simulink model "simu"  (R2023b)
settings: Solver=VariableStepAuto  StartTime=0.0  StopTime=1  RelTol=1e-3
values from neighbouring files (symbols this model uses):
  J = J_r+J_m+J_d    (= 2.15e-05)    [K_calculator.m]    (also in Velocity.m; mappe2.m)
  K_b = 0.042    [K_calculator.m]    (also in Velocity.m; mappe2.m)
  K_t = 0.042    [K_calculator.m]    (also in Velocity.m; mappe2.m)
  R_a = 8.4    [K_calculator.m]    (also in Velocity.m; mappe2.m)
settings Model: Creator=vegar  LastModifiedBy=vegar

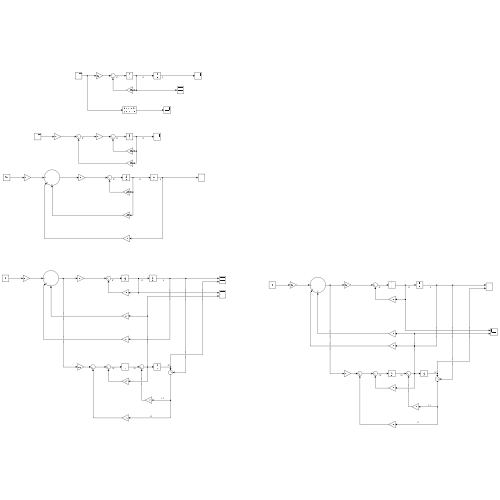
[thumbnail: Simulink's stored preview of the top-level diagram]
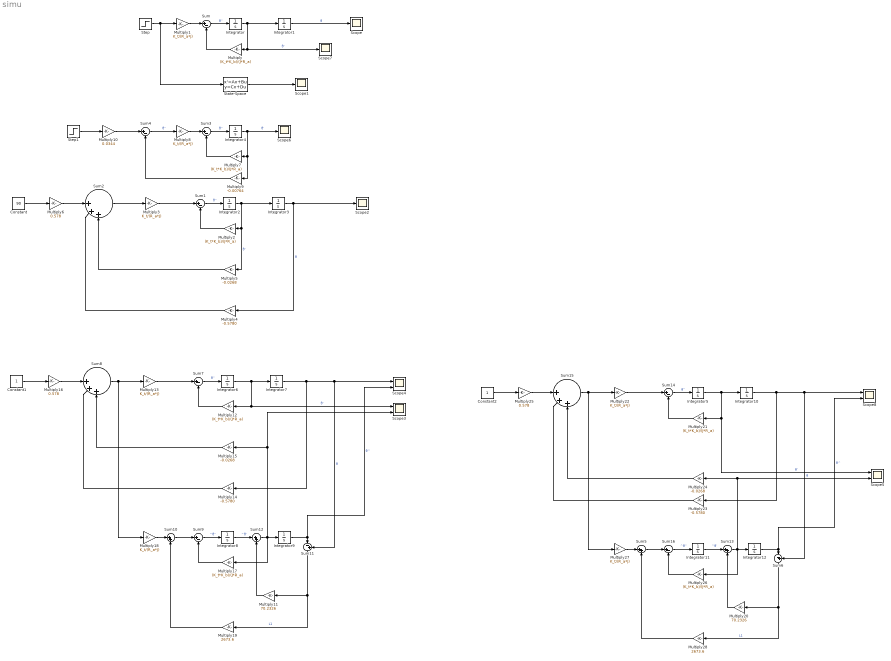
== system simu ==
  Constant : Constant  Value=90
  Constant1 : Constant
  Constant2 : Constant
  Integrator{,1..2,4..6,8..9,11..12} (10 alike) : Integrator
  Integrator10 : Integrator  InitialCondition=30
  Integrator3 : Integrator  InitialCondition=0.1
  Integrator7 : Integrator  InitialCondition=30
  Multiply{,2,7,12,17,21,26} (7 alike) : Gain  Gain=(K_t*K_b)/(J*R_a)
  Multiply{1,3,8,13,18,22,27} (7 alike) : Gain  Gain=K_t/(R_a*J)
  Multiply10 : Gain  Gain=0.0344
  Multiply11 : Gain  Gain=70.2326
  Multiply14 : Gain  Gain=-0.5780
  Multiply15 : Gain  Gain=-0.0268
  Multiply16 : Gain  Gain=0.578
  Multiply19 : Gain  Gain=2673.6
  Multiply20 : Gain  Gain=70.2326
  Multiply23 : Gain  Gain=-0.5780
  Multiply24 : Gain  Gain=-0.0268
  Multiply25 : Gain  Gain=0.578
  Multiply28 : Gain  Gain=2673.6
  Multiply4 : Gain  Gain=-0.5780
  Multiply5 : Gain  Gain=-0.0268
  Multiply6 : Gain  Gain=0.578
  Multiply9 : Gain  Gain=-0.00764
  Scope{,1..2,6..7} (5 alike) : Scope
  Scope{3..5,8} (4 alike) : Scope  NumInputPorts=2
  State-Space : StateSpace  A=[0 1; 0 -(K_t*K_b)/(J*R_a)]  B=[0;K_t/(R_a*J)]  C=[1 0]  D=0  InitialCondition=0
  Step : Step  SampleTime=0
  Step1 : Step  After=203  SampleTime=0
  Sum{,1,3..4,7,9,14,16} (8 alike) : Sum  Inputs=|+-
  Sum{5,10,12..13} (4 alike) : Sum  Inputs=|++
  Sum11 : Sum  Inputs=|-+
  Sum15 : Sum  Inputs=||+++
  Sum2 : Sum  Inputs=||+++
  Sum6 : Sum  Inputs=|-+
  Sum8 : Sum  Inputs=||+++
  wires:
  Integrator1/1 -> Scope/1  "θ"
  Integrator/1 -> Integrator1/1, Scope7/1, Multiply/1  "θ'"
  Sum/1 -> Integrator/1  "θ''"
  Step/1 -> Multiply1/1, State-Space/1
  Multiply/1 -> Sum/2
  State-Space/1 -> Scope1/1
  Sum1/1 -> Integrator2/1  "θ''"
  Multiply2/1 -> Sum1/2
  Integrator2/1 -> Multiply2/1, Multiply5/1, Integrator3/1  "θ'"
  Integrator3/1 -> Scope2/1, Multiply4/1  "θ"
  Multiply4/1 -> Sum2/2
  Multiply5/1 -> Sum2/3
  Constant/1 -> Multiply6/1
  Sum2/1 -> Multiply3/1
  Multiply6/1 -> Sum2/1
  Multiply3/1 -> Sum1/1
  Multiply19/1 -> Sum10/2
  Sum10/1 -> Sum9/1
  Multiply18/1 -> Sum10/1
  Multiply11/1 -> Sum12/2
  Sum11/1 -> Multiply11/1, Multiply19/1  "L1"
  Multiply13/1 -> Sum7/1
  Sum12/1 -> Multiply15/1, Scope3/2, Multiply17/1, Integrator9/1
  Multiply16/1 -> Sum8/1
  Integrator9/1 -> Scope4/2, Sum11/1  "θ^"
  Sum9/1 -> Integrator8/1  "^θ''"
  Integrator7/1 -> Scope4/1, Sum11/2, Multiply14/1  "θ"
  Integrator8/1 -> Sum12/1  "^θ'"
  Multiply12/1 -> Sum7/2
  Constant1/1 -> Multiply16/1
  Integrator6/1 -> Integrator7/1, Scope3/1, Multiply12/1  "θ'"
  Multiply14/1 -> Sum8/2
  Sum7/1 -> Integrator6/1  "θ''"
  Sum8/1 -> Multiply18/1, Multiply13/1
  Multiply17/1 -> Sum9/2
  Multiply15/1 -> Sum8/3
  Multiply1/1 -> Sum/1
  Multiply7/1 -> Sum3/2
  Multiply8/1 -> Sum3/1
  Sum3/1 -> Integrator4/1  "θ''"
  Integrator4/1 -> Scope6/1, Multiply9/1, Multiply7/1  "θ'"
  Sum4/1 -> Multiply8/1  "θ''"
  Multiply9/1 -> Sum4/2
  Step1/1 -> Multiply10/1
  Multiply10/1 -> Sum4/1
  Integrator11/1 -> Sum13/1  "^θ'"
  Multiply20/1 -> Sum13/2
  Sum13/1 -> Multiply26/1, Multiply24/1, Scope5/2, Integrator12/1
  Multiply25/1 -> Sum15/1
  Sum5/1 -> Sum16/1
  Sum15/1 -> Multiply27/1, Multiply22/1
  Multiply21/1 -> Sum14/2
  Multiply24/1 -> Sum15/3
  Integrator12/1 -> Scope8/2, Sum6/1  "θ^"
  Multiply22/1 -> Sum14/1
  Constant2/1 -> Multiply25/1
  Sum16/1 -> Integrator11/1  "^θ''"
  Multiply23/1 -> Sum15/2
  Multiply28/1 -> Sum5/2
  Multiply27/1 -> Sum5/1
  Sum6/1 -> Multiply20/1, Multiply28/1  "L1"
  Multiply26/1 -> Sum16/2
  Integrator5/1 -> Integrator10/1, Scope5/1, Multiply21/1  "θ'"
  Integrator10/1 -> Scope8/1, Sum6/2, Multiply23/1  "θ"
  Sum14/1 -> Integrator5/1  "θ''"
